simulink model "hw1_1"  (R2019a)
settings: Solver=FixedStepAuto  StartTime=0.0  StopTime=50  FixedStep=0.001  RelTol=1e-3
settings Model: Creator=hebuyong  LastModifiedBy=hebuyong

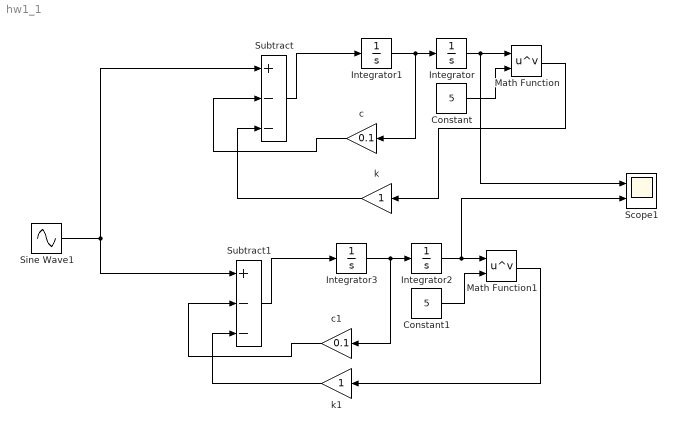
== system hw1_1 ==
  Constant : Constant  Value=5
  Constant1 : Constant  Value=5
  Integrator : Integrator  InitialCondition=2
  Integrator1 : Integrator  InitialCondition=3
  Integrator2 : Integrator  InitialCondition=2.01
  Integrator3 : Integrator  InitialCondition=3.01
  Math Function : Math  Operator=pow  SaturateOnIntegerOverflow=on
  Math Function1 : Math  Operator=pow  SaturateOnIntegerOverflow=on
  Scope1 : Scope  NumInputPorts=2
  Sine Wave1 : Sin  Amplitude=6  SampleTime=0
  Subtract : Sum  Inputs=+--
  Subtract1 : Sum  Inputs=+--
  c : Gain  Gain=0.1
  c1 : Gain  Gain=0.1
  k : Gain
  k1 : Gain
  wires:
  Integrator/1 -> Scope1/1, Math Function/1
  Integrator1/1 -> c/1, Integrator/1
  c/1 -> Subtract/2
  Math Function/1 -> k/1
  k/1 -> Subtract/3
  Subtract/1 -> Integrator1/1
  Constant/1 -> Math Function/2
  Constant1/1 -> Math Function1/2
  Integrator3/1 -> c1/1, Integrator2/1
  Integrator2/1 -> Scope1/2, Math Function1/1
  Sine Wave1/1 -> Subtract1/1, Subtract/1
  k1/1 -> Subtract1/3
  Math Function1/1 -> k1/1
  Subtract1/1 -> Integrator3/1
  c1/1 -> Subtract1/2
